simulink model "es1_simulink"  (R2022a)
settings: Solver=VariableStepAuto  StartTime=0.0  StopTime=3  RelTol=1e-3
values from neighbouring files (symbols this model uses):
  Cd = c2d(C,Tc,'tustin')    [es1.m]
  G = tf(num,den)    [es1.m]
  Tc = 0.001    [es1.m]
settings Model: Creator=Stefano  LastModifiedBy=Stefano

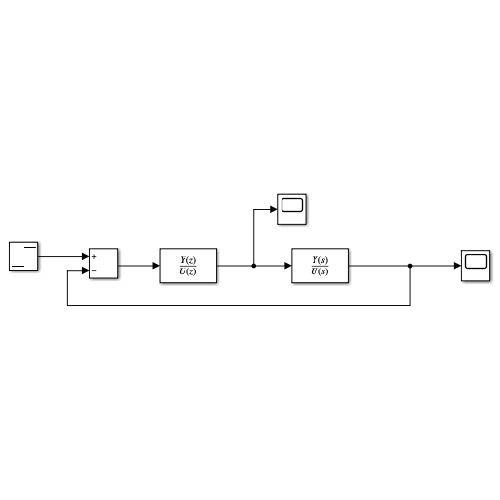
[thumbnail: Simulink's stored preview of the top-level diagram]
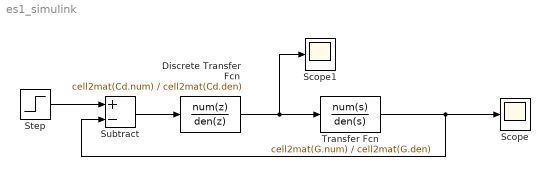
== system es1_simulink ==
  Discrete Transfer Fcn : DiscreteTransferFcn  Numerator=cell2mat(Cd.num)  Denominator=cell2mat(Cd.den)  SampleTime=Tc
  Scope : Scope
  Scope1 : Scope
  Step : Step  SampleTime=0
  Subtract : Sum  Inputs=+-
  Transfer Fcn : TransferFcn  Numerator=cell2mat(G.num)  Denominator=cell2mat(G.den)
  wires:
  Discrete Transfer Fcn/1 -> Scope1/1, Transfer Fcn/1
  Step/1 -> Subtract/1
  Subtract/1 -> Discrete Transfer Fcn/1
  Transfer Fcn/1 -> Subtract/2, Scope/1
